simulink model "AOO"  (R2022a)
settings: Solver=FixedStepAuto  StartTime=0.0  StopTime=10.0  FixedStep=1e-3  RelTol=1e-3  EnableMultiTasking=on
undefined symbols (not defined in the file): D3, PTA1
libraries: frdmk64flib x1
settings Model: ExtModeTrigDuration=5  Creator=Aldraech  LastModifiedBy=Aldraech
settings OptimizationCC: EnhancedBackFolding=on  PassReuseOutputArgsAs=Individual arguments  ZeroExternalMemoryAtStartup=off  ZeroInternalMemoryAtStartup=off  MaxStackSize=64  OptimizeBlockOrder=speed  DifferentSizesBufferReuse=on  OptimizationCustomize=off  EfficientTunableParamExpr=on
settings DebuggingCC: ParameterTunabilityLossMsg=error
settings HardwareCC: ProdBitPerPointer=32  ProdBitPerSizeT=32  ProdBitPerPtrDiffT=32  ProdLargestAtomicInteger=Long  ProdLargestAtomicFloat=Double  ProdWordSize=32  ProdHWDeviceType=ARM Compatible->ARM Cortex
settings SFSimCC: MATLABDynamicMemAlloc=off
settings RTWCC: SystemTargetFile=ert.tlc  HardwareBoard=NXP FRDM-K64F  TLCOptions="-aInlineSetEventsForThisBaseRateFcn=TLC_FALSE -aSuppressMultiTaskScheduler=TLC_FALSE  -aRateBasedStepFcn=0"  TemplateMakefile=ert_default_tmf  Toolchain=GNU Tools for ARM Embedded Processors
settings CodeAppCC: ForceParamTrailComments=on  IgnoreCustomStorageClasses=off  OperatorAnnotations=on  SimulinkDataObjDesc=on  SFDataObjDesc=on  InsertBlockDesc=on
settings ERTTargetCC: ExtModeTransport=4  ExtModeMexFile=sendToCommService

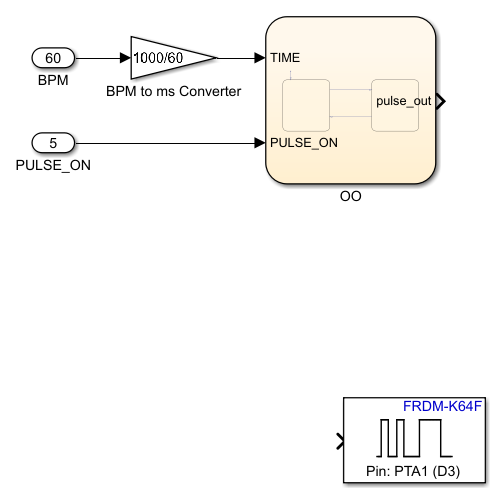
[thumbnail: Simulink's stored preview of the top-level diagram]
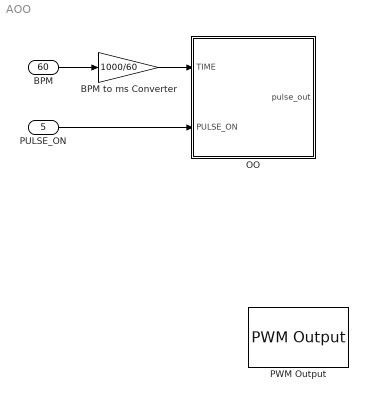
== system AOO ==
  PULSE_ON : Inport  Port=5
  BPM : Inport  Port=60
  BPM to ms Converter : Gain  Gain=1000/60
  OO : Stateflow chart  TreatAsAtomicUnit=on
  PWM Output : frdmk64flib/PWM Output  Whichpin=PTA1 (D3)  InitialFrequency=2000  InitialDutyCycle=20
  wires:
  BPM/1 -> BPM to ms Converter/1
  PULSE_ON/1 -> OO/2(PULSE_ON)
  BPM to ms Converter/1 -> OO/1(TIME)

== stateflow chart AOO/OO ==
  state Charge
    entry:
    TIME = TIME - PULSE_ON
    pulse_out = 0
  state Generate_Pulse
    entry:
    pulse_out = 1
  (default) -> Charge
  Charge -> Generate_Pulse : after(TIME, msec)
  Generate_Pulse -> Charge : after(PULSE_ON, msec)
  data: pulse_out output; TIME input; PULSE_ON input
